simulink model "MUL_IFF_NON_LIN"  (R2022b)
settings: Solver=VariableStepAuto  StartTime=0.0  StopTime=40  RelTol=1e-3
model workspace (MATLAB code in the model file):
  | Kia=5;
  | Fa=8;
  | Kba=8;
  | Fb=6;
  | Kcb=8;
  | Fc=4;
  | Kdc=8;
  | Fd=5;
  | Keb=8;
  | Ked=8;
  | In=0.3;
  | x_star=[0.1875; 0.250; 0.5000; 0.8000; 0.3125];
settings Model: Creator=priya  LastModifiedBy=pxb271
settings SolverCC: AlgebraicLoopSolver=TrustRegion
settings DebuggingCC: UnconnectedInputMsg=warning  UnconnectedOutputMsg=warning  UnconnectedLineMsg=warning  SFMachineParentedDataDiag=warning
settings ModelReferenceCC: EnableRefExpFcnMdlSchedulingChecks=on
settings RTWCC: DLArmComputeVersion=19.05

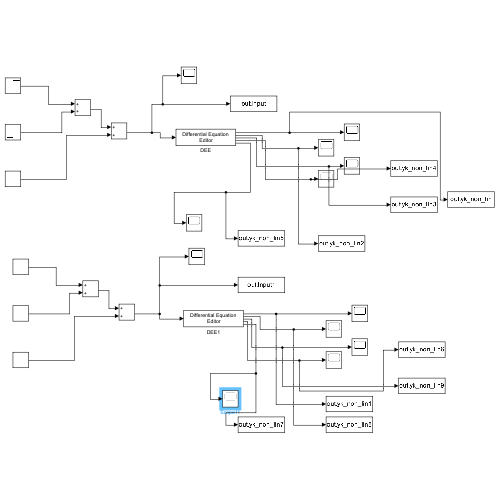
[thumbnail: Simulink's stored preview of the top-level diagram]
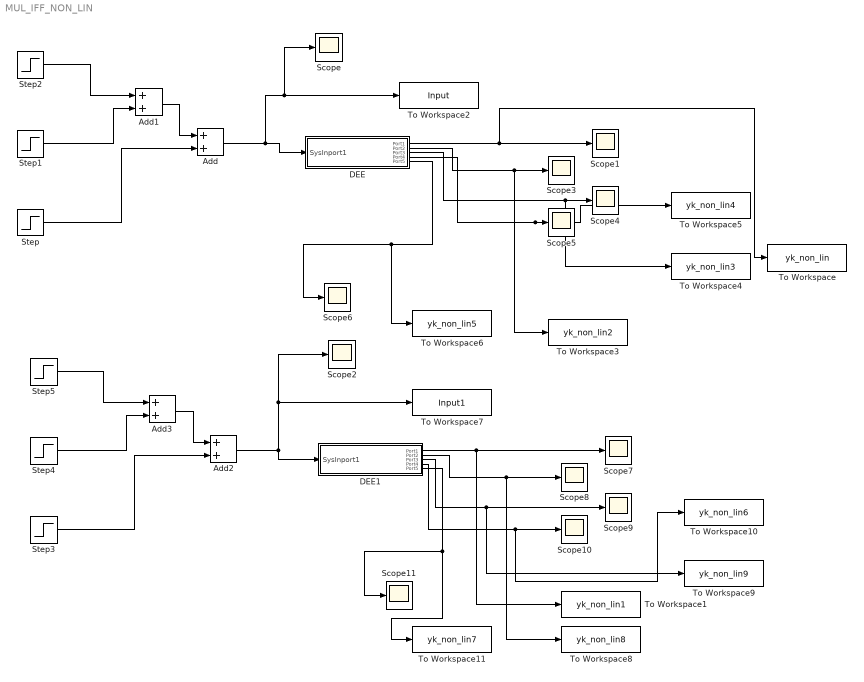
== system MUL_IFF_NON_LIN ==
  Add : Sum  OutDataTypeStr=Inherit: Keep MSB
  Add1 : Sum
  Add2 : Sum  OutDataTypeStr=Inherit: Keep MSB
  Add3 : Sum
  DEE : Subsystem  mask(Differential Equation Editor (DEE)){}
      settings: OpenFcn=diffeqed
      mask Display: disp('Differential Equation\n Editor')
  DEE1 : Subsystem  mask(Differential Equation Editor (DEE)){}
      settings: OpenFcn=diffeqed
      mask Display: disp('Differential Equation\n Editor')
  Scope{,1..11} (12 alike) : Scope
  Step : Step  Time=20  After=40  SampleTime=0
  Step1 : Step  Time=10  After=30  SampleTime=0
  Step2 : Step  Time=0  After=15  SampleTime=0
  Step3 : Step  Time=20  After=40  SampleTime=0
  Step4 : Step  Time=10  After=30  SampleTime=0
  Step5 : Step  Time=0  After=15  SampleTime=0
  To Workspace : ToWorkspace  VariableName=yk_non_lin  SampleTime=-1
  To Workspace1 : ToWorkspace  VariableName=yk_non_lin1  SampleTime=-1
  To Workspace10 : ToWorkspace  VariableName=yk_non_lin6  SampleTime=-1
  To Workspace11 : ToWorkspace  VariableName=yk_non_lin7  SampleTime=-1
  To Workspace2 : ToWorkspace  VariableName=Input  SampleTime=-1
  To Workspace3 : ToWorkspace  VariableName=yk_non_lin2  SampleTime=-1
  To Workspace4 : ToWorkspace  VariableName=yk_non_lin3  SampleTime=-1
  To Workspace5 : ToWorkspace  VariableName=yk_non_lin4  SampleTime=-1
  To Workspace6 : ToWorkspace  VariableName=yk_non_lin5  SampleTime=-1
  To Workspace7 : ToWorkspace  VariableName=Input1  SampleTime=-1
  To Workspace8 : ToWorkspace  VariableName=yk_non_lin8  SampleTime=-1
  To Workspace9 : ToWorkspace  VariableName=yk_non_lin9  SampleTime=-1
  wires:
  Step2/1 -> Add1/1
  Step1/1 -> Add1/2
  Add1/1 -> Add/1
  Step/1 -> Add/2
  Add/1 -> DEE/1(SysInport1), To Workspace2/1, Scope/1
  DEE/1(Port1) -> To Workspace/1, Scope1/1
  DEE/2(Port2) -> To Workspace3/1, Scope3/1
  DEE/3(Port3) -> To Workspace4/1, Scope4/1
  DEE/4(Port4) -> To Workspace5/1, Scope5/1
  DEE/5(Port5) -> To Workspace6/1, Scope6/1
  DEE1/5(Port5) -> To Workspace11/1, Scope11/1
  DEE1/3(Port3) -> To Workspace9/1, Scope9/1
  DEE1/2(Port2) -> To Workspace8/1, Scope8/1
  Add3/1 -> Add2/1
  Step4/1 -> Add3/2
  DEE1/1(Port1) -> To Workspace1/1, Scope7/1
  Add2/1 -> DEE1/1(SysInport1), To Workspace7/1, Scope2/1
  DEE1/4(Port4) -> To Workspace10/1, Scope10/1
  Step3/1 -> Add2/2
  Step5/1 -> Add3/1

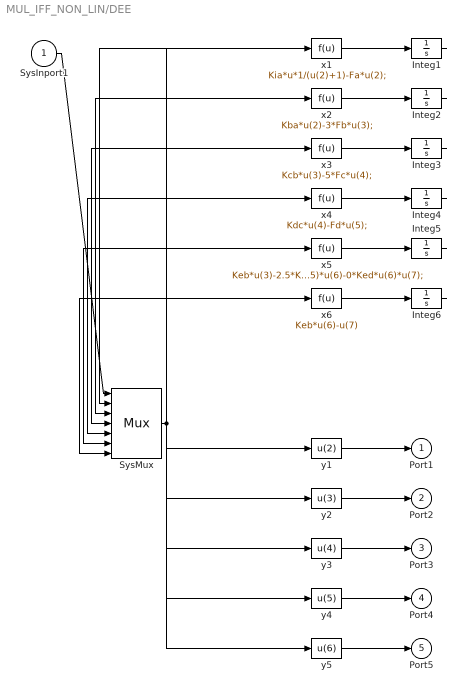
== system MUL_IFF_NON_LIN/DEE ==
  SysInport1 : Inport
  Integ1 : Integrator  InitialCondition=x_star(1)
  Integ2 : Integrator  InitialCondition=x_star(2)
  Integ3 : Integrator  InitialCondition=x_star(3)
  Integ4 : Integrator  InitialCondition=x_star(4)
  Integ5 : Integrator  InitialCondition=0.5*x_star(5)
  Integ6 : Integrator
  SysMux : Mux  Inputs=7
  x1 : Fcn  Expr=Kia*u*1/(u(2)+1)-Fa*u(2);
  x2 : Fcn  Expr=Kba*u(2)-3*Fb*u(3);
  x3 : Fcn  Expr=Kcb*u(3)-5*Fc*u(4);
  x4 : Fcn  Expr=Kdc*u(4)-Fd*u(5);
  x5 : Fcn  Expr=Keb*u(3)-2.5*Ked*u(5)*u(6)-0*Ked*u(6)*u(7);
  x6 : Fcn  Expr=Keb*u(6)-u(7)
  y1 : Fcn  Expr=u(2)
  y2 : Fcn  Expr=u(3)
  y3 : Fcn  Expr=u(4)
  y4 : Fcn  Expr=u(5)
  y5 : Fcn  Expr=u(6)
  Port1 : Outport
  Port2 : Outport  Port=2
  Port3 : Outport  Port=3
  Port4 : Outport  Port=4
  Port5 : Outport  Port=5
  wires:
  SysInport1/1 -> SysMux/1
  SysMux/1 -> x1/1, x2/1, x3/1, x4/1, x5/1, x6/1, y1/1, y2/1, y3/1, y4/1, y5/1
  x1/1 -> Integ1/1
  Integ1/1 -> SysMux/2
  x2/1 -> Integ2/1
  Integ2/1 -> SysMux/3
  x3/1 -> Integ3/1
  Integ3/1 -> SysMux/4
  x4/1 -> Integ4/1
  Integ4/1 -> SysMux/5
  x5/1 -> Integ5/1
  Integ5/1 -> SysMux/6
  x6/1 -> Integ6/1
  Integ6/1 -> SysMux/7
  y1/1 -> Port1/1
  y2/1 -> Port2/1
  y3/1 -> Port3/1
  y4/1 -> Port4/1
  y5/1 -> Port5/1

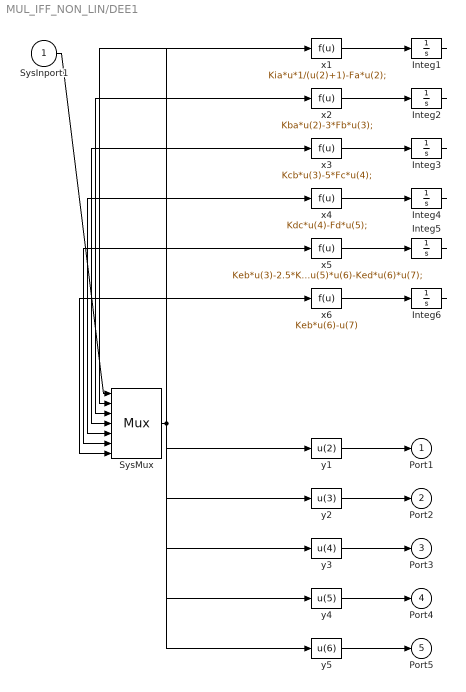
== system MUL_IFF_NON_LIN/DEE1 ==
  SysInport1 : Inport
  Integ1 : Integrator  InitialCondition=x_star(1)
  Integ2 : Integrator  InitialCondition=x_star(2)
  Integ3 : Integrator  InitialCondition=x_star(3)
  Integ4 : Integrator  InitialCondition=x_star(4)
  Integ5 : Integrator  InitialCondition=0.5*x_star(5)
  Integ6 : Integrator
  SysMux : Mux  Inputs=7
  x1 : Fcn  Expr=Kia*u*1/(u(2)+1)-Fa*u(2);
  x2 : Fcn  Expr=Kba*u(2)-3*Fb*u(3);
  x3 : Fcn  Expr=Kcb*u(3)-5*Fc*u(4);
  x4 : Fcn  Expr=Kdc*u(4)-Fd*u(5);
  x5 : Fcn  Expr=Keb*u(3)-2.5*Ked*u(5)*u(6)-Ked*u(6)*u(7);
  x6 : Fcn  Expr=Keb*u(6)-u(7)
  y1 : Fcn  Expr=u(2)
  y2 : Fcn  Expr=u(3)
  y3 : Fcn  Expr=u(4)
  y4 : Fcn  Expr=u(5)
  y5 : Fcn  Expr=u(6)
  Port1 : Outport
  Port2 : Outport  Port=2
  Port3 : Outport  Port=3
  Port4 : Outport  Port=4
  Port5 : Outport  Port=5
  wires:
  SysInport1/1 -> SysMux/1
  SysMux/1 -> x1/1, x2/1, x3/1, x4/1, x5/1, x6/1, y1/1, y2/1, y3/1, y4/1, y5/1
  x1/1 -> Integ1/1
  Integ1/1 -> SysMux/2
  x2/1 -> Integ2/1
  Integ2/1 -> SysMux/3
  x3/1 -> Integ3/1
  Integ3/1 -> SysMux/4
  x4/1 -> Integ4/1
  Integ4/1 -> SysMux/5
  x5/1 -> Integ5/1
  Integ5/1 -> SysMux/6
  x6/1 -> Integ6/1
  Integ6/1 -> SysMux/7
  y1/1 -> Port1/1
  y2/1 -> Port2/1
  y3/1 -> Port3/1
  y4/1 -> Port4/1
  y5/1 -> Port5/1
